simulink subsystem "subsystem_disturbanceObserver"  (R2022a)
settings: Solver=VariableStepAuto  StartTime=0.0  StopTime=10.0  RelTol=1e-3
settings Model: Creator=Philipp  LastModifiedBy=Philipp
settings DebuggingCC: UnconnectedInputMsg=warning  UnconnectedOutputMsg=warning  UnconnectedLineMsg=warning
settings RTWCC: DLArmComputeVersion=19.05

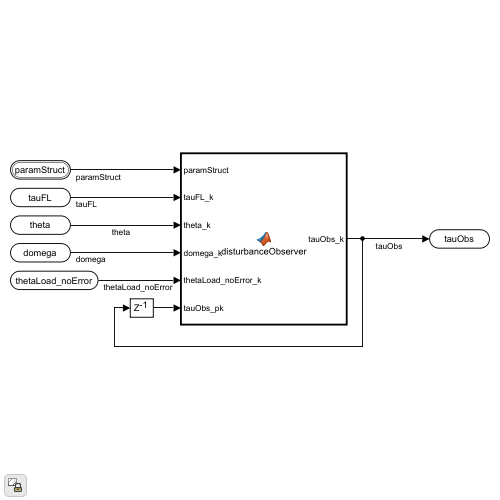
[thumbnail: Simulink's stored preview of the top-level diagram]
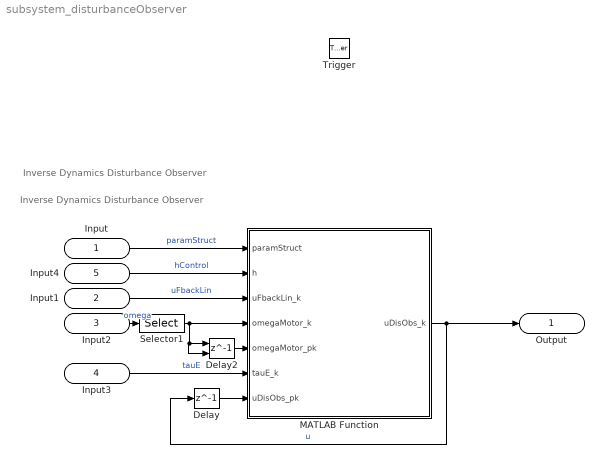
== system subsystem_disturbanceObserver ==
  note: Inverse Dynamics Disturbance Observer
  note: Inverse Dynamics Disturbance Observer
  Input : Inport  OutDataTypeStr=Bus: main_bus
  Input1 : Inport  Port=2
  Input2 : Inport  Port=3
  Input3 : Inport  Port=4
  Input4 : Inport  Port=5
  Trigger : TriggerPort  VariantControl=(inherit)
  Delay : Delay  DelayLength=1
  Delay2 : Delay  DelayLength=1  InitialConditionSource=Input port
      settings: InputPortMap=u0,p4
  MATLAB Function : MATLAB Function  TreatAsAtomicUnit=on
  Selector1 : Selector  InputPortWidth=6  IndexOptions=Index vector (dialog)  Indices=4:6  OutputSizes=1
  Output : Outport
  wires:
  MATLAB Function/1(uDisObs_k) -> Delay/1, Output/1  "u"
  Input/1 -> MATLAB Function/1(paramStruct)  "paramStruct"
  Input3/1 -> MATLAB Function/6(tauE_k)  "tauE"
  Input2/1 -> Selector1/1  "omega"
  Input4/1 -> MATLAB Function/2(h)  "hControl"
  Input1/1 -> MATLAB Function/3(uFbackLin_k)  "uFbackLin"
  Delay2/1 -> MATLAB Function/5(omegaMotor_pk)
  Selector1/1 -> Delay2/2, Delay2/1, MATLAB Function/4(omegaMotor_k)
  Delay/1 -> MATLAB Function/7(uDisObs_pk)

== matlab function subsystem_disturbanceObserver/MATLAB Function ==
  data: paramStruct input; h input; uDisObs_k output; uFbackLin_k input; omegaMotor_k input; omegaMotor_pk input; tauE_k input; uDisObs_pk input
function uDisObs_k  = disturbanceObserver(paramStruct, h, uFbackLin_k, omegaMotor_k, omegaMotor_pk, tauE_k, uDisObs_pk)

uDisObs_k = disturbanceObserver_model(paramStruct, h, uFbackLin_k, omegaMotor_k, omegaMotor_pk, tauE_k, uDisObs_pk);
